simulink model "main_temp_new"  (R2021b)
settings: Solver=VariableStepAuto  StartTime=0.0  StopTime=50  RelTol=1e-3
model workspace (MAT data in the model file):
  op_trim2 : opcond.OperatingReport (value not decoded)
values from neighbouring files (symbols this model uses):
  ail = 8.316800428880180e-15    (= 8.31680042888e-15)    [lookupdata.m]
  CL = [  .0     .0     .0     .0     .0     .0     .0     .0     .0     .0     .0     .0 ... (first row only)    [lookupdata.m]
  CL2 = [ -.041  -.052  -.053  -.056  -.050  -.056  -.082  -.059  -.042  -.038  -.027  -.017 ... (first row only)    [lookupdata.m]
  CL3 = [ .005  .017  .014  .010  -.005  .009  .019  .005   .000  -.005  -.011  .008 ... (first row only)    [lookupdata.m]
  CLp = Damp(6,:)    [lookupdata.m]
  CLr = Damp(5,:)    [lookupdata.m]
  CM = [ .205   .168   .186   .196   .213   .251   .245   .238   .252   .231   .198   .192 ... (first row only)    [lookupdata.m]
  CMq = Damp(7,:)    [lookupdata.m]
  CN = [ .0    .0    .0    .0    .0    .0    .0    .0    .0     .0     .0     .0 ... (first row only)    [lookupdata.m]
  CN2 = [  .001  -.027  -.017  -.013  -.012  -.016   .001   .017   .011  .017   .008  .016 ... (first row only)    [lookupdata.m]
  CN3 = [ -.018  -.052  -.052  -.052  -.054  -.049  -.059  -.051  -.030  -.037  -.026  -.013 ... (first row only)    [lookupdata.m]
  CNp = Damp(9,:)    [lookupdata.m]
  CNr = Damp(8,:)    [lookupdata.m]
  CX = [ -0.0990   -0.0480   -0.0220   -0.0400   -0.0830 ... (first row only)    [lookupdata.m]
  CXq = Damp(1,:)    [lookupdata.m]
  CYp = Damp(3,:)    [lookupdata.m]
  CYr = Damp(2,:)    [lookupdata.m]
  CZ = [ 0.770  0.241  -0.100  -0.416  -0.731  -1.053  -1.366                                  -1.646  -1.917  -2.120  -2.248  -2.229 ]    [lookupdata.m]
  CZq = Damp(4,:)    [lookupdata.m]
  el = -2.205494777225563    (= -2.20549477723)    [lookupdata.m]
  Klqrlat = lqr(sys,Q,R)    [lat_lqr.m]
  Klqrlong = lqr(sys,Q,R)    [long_lqr.m]
  rud = -6.804083993307187e-14    (= -6.80408399331e-14)    [lookupdata.m]
  state_init = [ 598.9416 ; 0 ; 35.622639 ; 0 ; 0 ; 0 ;  0.01  ; 0.1 ;  0.1  ;        0 ; 0 ; 19950 ; 590 ; 0.059405952482911 ; 0 ; 15.941298293587984]    [lookupdata.m]
  th = 0.245477337443609    (= 0.245477337444)    [lookupdata.m]
  x_lat = [   0   ;     0    ;  0  ;  0  ; 0]    [lookupdata.m]
  x_long = [600 ; 20000 ; 0.059405952482911 ; 0.059405952482911 ; 0 ; 15.941298293587984]    [lookupdata.m]
undefined symbols (not defined in the file or in its folder): Earth, WGS84
libraries: simulink x4, aerolibfltsims x2, aerolibtransform2 x1, sldrtlib x1
settings Model: Creator=TecHNo-Pc  LastModifiedBy=TecHNo-Pc
settings SolverCC: AlgebraicLoopSolver=TrustRegion
settings DataIOCC: ExternalInput=getinputstruct(op_trim2)  InitialState=state_init  LoadInitialState=on
settings DebuggingCC: SFMachineParentedDataDiag=warning

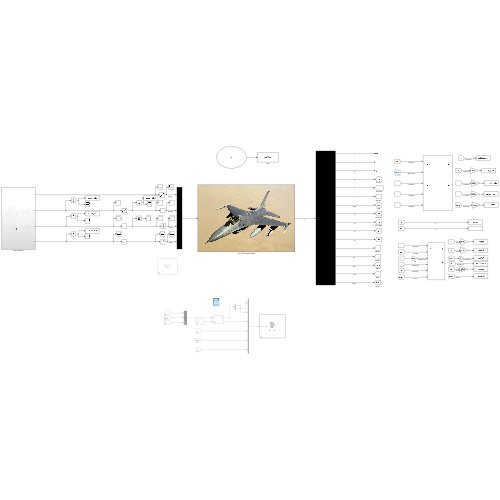
[thumbnail: Simulink's stored preview of the top-level diagram]
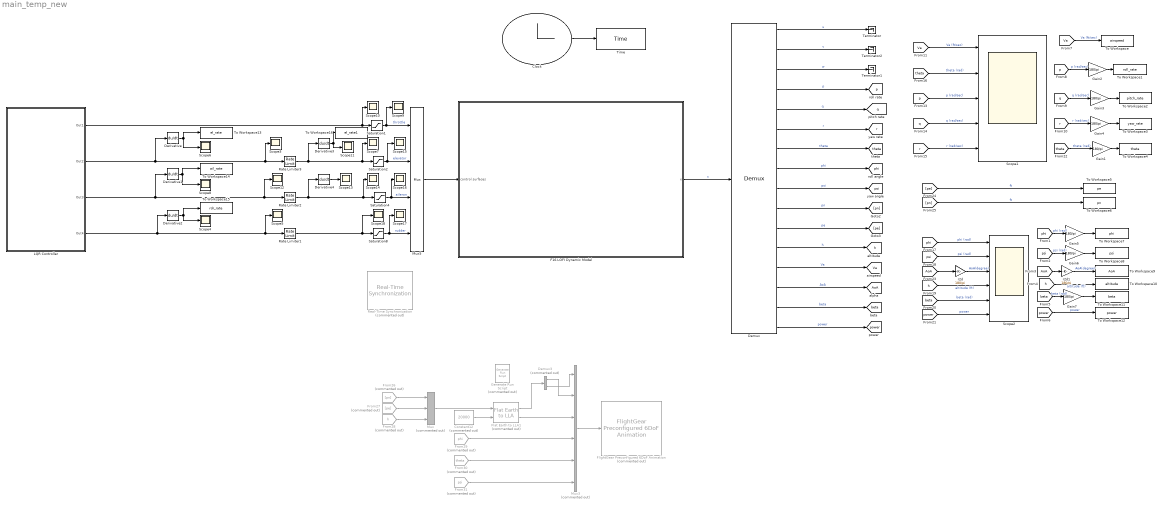
== system main_temp_new ==
  Clock : Clock
      settings: Decimation=50
  Constant12 : Constant  Commented=on  Value=20000
  Demux : Demux  Outputs=16
  Demux3 : Demux  Commented=on  Outputs=2
  Derivative{,1..4} (5 alike) : Derivative
  F16 LOFI Dynamic Model : Subsystem
      mask Display: image('$imagefile'); % Use "Edit Image" on toolstrip to change.
  Flat Earth to LLA1 : aerolibtransform2/Flat Earth to LLA  Commented=on  units=English  ptype=Earth (WGS84)  F=1/298.257223563  R=20925646.3255  refPosPort=off  LL0=[0 10]  psi=0
  FlightGear Preconfigured 6DoF Animation : aerolibfltsims/FlightGear Preconfigured 6DoF Animation  Commented=on  xFlightGearVersion=v2019.1  DestinationIpAddress=127.0.0.1  DestinationPort=5502  SampleTime=1/30  packetVersion=24
  From26 : From  Commented=on  GotoTag=pn
  From27 : From  Commented=on  GotoTag=pe
  From28 : From  Commented=on  GotoTag=h  TagVisibility=global
  From29 : From  Commented=on  GotoTag=phi  TagVisibility=global
  From30 : From  Commented=on  GotoTag=theta  TagVisibility=global
  From31 : From  Commented=on  GotoTag=psi  TagVisibility=global
  Gain{1..7} (7 alike) : Gain  Gain=180/pi
  Generate Run Script : aerolibfltsims/Generate Run Script  Commented=on  Architecture=Default  dataFlow=Send  GeometryModelName=c172p  AirportId=KSFO  RunwayId=10L  InitialAltitude=7224  InitialHeading=113  OffsetDistance=4.72  OffsetAzimuth=0  InstallScenery=off  DisableShaders=off  OriginAddress=127.0.0.1  DestinationPort=5502  OriginPort=5505  LocalAddress=127.0.0.1  OutputFileName=runfg.bat  FlightGearBaseDirectory=C:\Program Files\FlightGear 2020.3
  LQR Controller : Subsystem
  Mux : Mux  Commented=on  Inputs=3
  Mux3 : Mux  Commented=on  Inputs=6
  Mux5 : Mux
  Rate Limiter1 : RateLimiter  RisingSlewLimit=120  FallingSlewLimit=-120  SampleTimeMode=inherited
  Rate Limiter2 : RateLimiter  RisingSlewLimit=80  FallingSlewLimit=-80  SampleTimeMode=inherited
  Rate Limiter3 : RateLimiter  RisingSlewLimit=60  FallingSlewLimit=-60  SampleTimeMode=inherited
  Real-Time Synchronization : sldrtlib/Real-Time Synchronization  Commented=on  SampleTime=0.1  MaxMissedTicks=10  ShowMissedTicks=off  YieldWhenWaiting=off
  Saturation1 : Saturate  UpperLimit=1  LowerLimit=0
  Saturation2 : Saturate  UpperLimit=25  LowerLimit=-25
  Saturation4 : Saturate  UpperLimit=21.5  LowerLimit=-21.5
  Saturation8 : Saturate  UpperLimit=30  LowerLimit=-30
  Scope1 : Scope  NumInputPorts=5
  Scope{3..18} (16 alike) : Scope
  Scope2 : Scope  NumInputPorts=6
  Terminator : Terminator
  Terminator1 : Terminator
  Terminator2 : Terminator
  Time : ToWorkspace  VariableName=Time  SampleTime=-1
      settings: Decimation=100
  To Workspace : ToWorkspace  VariableName=airspeed  SampleTime=-1
  To Workspace1 : ToWorkspace  VariableName=roll_rate  SampleTime=-1
  To Workspace10 : ToWorkspace  VariableName=altitude  SampleTime=-1
  To Workspace11 : ToWorkspace  VariableName=beta  SampleTime=-1
  To Workspace12 : ToWorkspace  VariableName=power  SampleTime=-1
  To Workspace13 : ToWorkspace  VariableName=el_rate  SampleTime=-1
  To Workspace14 : ToWorkspace  VariableName=ail_rate  SampleTime=-1
  To Workspace15 : ToWorkspace  VariableName=rdr_rate  SampleTime=-1
  To Workspace16 : ToWorkspace  VariableName=el_rate1  SampleTime=-1
  To Workspace2 : ToWorkspace  VariableName=pitch_rate  SampleTime=-1
  To Workspace3 : ToWorkspace  VariableName=yaw_rate  SampleTime=-1
  To Workspace4 : ToWorkspace  VariableName=theta  SampleTime=-1
  To Workspace5 : ToWorkspace  VariableName=pe  SampleTime=-1
  To Workspace6 : ToWorkspace  VariableName=pn  SampleTime=-1
  To Workspace7 : ToWorkspace  VariableName=phi  SampleTime=-1
  To Workspace8 : ToWorkspace  VariableName=psi  SampleTime=-1
  To Workspace9 : ToWorkspace  VariableName=AoA  SampleTime=-1
  r2d : Gain  Gain=180/pi
  r2d1 : Gain  Gain=180/pi
  tag scope: AoA=global, Va=global, beta=global, h=global, p=global, phi=global, power=global, psi=global, q=global, r=global, theta=global
  wires:
  Demux/2 -> Terminator2/1  "v"
  Demux/3 -> Terminator1/1  "w"
  Demux/4 -> [p]  "p"
  Demux/6 -> [r]  "r"
  Demux/7 -> [theta]  "theta"
  Demux/8 -> [phi]  "phi"
  Demux/9 -> [psi]  "psi"
  Demux/10 -> [pn]  "pn"
  Demux/11 -> [pe]  "pe"
  Mux5/1 -> F16 LOFI Dynamic Model/1(control surfaces)
  Demux/13 -> [Va]  "Va"
  Demux/14 -> [AoA]  "AoA"
  Demux/15 -> [beta]  "beta"
  Demux/16 -> [power]  "power"
  Demux/1 -> Terminator/1  "u"
  Demux/5 -> [q]  "q"
  Demux/12 -> [h]  "h"
  F16 LOFI Dynamic Model/1(x) -> Demux/1  "x"
  [Va] -> Scope1/1  "Va (ft/sec)"
  [p] -> Scope1/3  "p (rad/sec)"
  [q] -> Scope1/4  "q (rad/sec)"
  [r] -> Scope1/5  "r (rad/sec)"
  [theta] -> Scope1/2  "theta (rad)"
  [phi] -> Scope2/1  "phi (rad)"
  [psi] -> Scope2/2  "psi (rad)"
  r2d/1 -> Scope2/3  "AoA(degree)"
  [h] -> Scope2/4  "altitude (ft)"
  [beta] -> Scope2/5  "beta (rad)"
  [power] -> Scope2/6  "power"
  [AoA] -> r2d/1
  [pe] -> To Workspace5/1  "ft"
  [pn] -> To Workspace6/1  "ft"
  Clock/1 -> Time/1
  Constant12/1 -> Flat Earth to LLA1/2
  Demux3/2 -> Mux3/1
  Demux3/1 -> Mux3/2
  Flat Earth to LLA1/1 -> Demux3/1
  Mux3/1 -> FlightGear Preconfigured 6DoF Animation/1
  Flat Earth to LLA1/2 -> Mux3/3
  Mux/1 -> Flat Earth to LLA1/1
  From26/1 -> Mux/1
  From27/1 -> Mux/2
  From28/1 -> Mux/3
  From29/1 -> Mux3/4
  From30/1 -> Mux3/5
  From31/1 -> Mux3/6
  Saturation2/1 -> Scope15/1, Mux5/2  "elevator"
  Saturation1/1 -> Scope9/1, Mux5/1  "throttle"
  Saturation4/1 -> Scope16/1, Mux5/3  "aileron"
  Saturation8/1 -> Scope17/1, Mux5/4  "rudder"
  LQR Controller/1(Out1) -> Saturation1/1, Scope10/1
  Gain1/1 -> To Workspace4/1
  Gain2/1 -> To Workspace1/1
  Gain3/1 -> To Workspace2/1
  Gain4/1 -> To Workspace3/1
  Gain5/1 -> To Workspace7/1
  Gain6/1 -> To Workspace8/1
  Gain7/1 -> To Workspace11/1
  Derivative/1 -> To Workspace13/1, Scope6/1
  LQR Controller/2(Out2) -> Rate Limiter3/1, Scope3/1, Derivative/1
  [phi] -> Gain5/1  "phi (rad)"
  [psi] -> Gain6/1  "psi (rad)"
  [AoA] -> r2d1/1
  r2d1/1 -> To Workspace9/1  "AoA(degree)"
  [beta] -> Gain7/1  "beta (rad)"
  [h] -> To Workspace10/1  "altitude (ft)"
  [power] -> To Workspace12/1  "power"
  [Va] -> To Workspace/1  "Va (ft/sec)"
  [p] -> Gain2/1  "p (rad/sec)"
  [q] -> Gain3/1  "q (rad/sec)"
  [r] -> Gain4/1  "r (rad/sec)"
  [theta] -> Gain1/1  "theta (rad)"
  Rate Limiter3/1 -> Derivative3/1, Scope7/1, Saturation2/1
  LQR Controller/3(Out3) -> Derivative1/1, Scope12/1, Rate Limiter2/1
  Derivative1/1 -> To Workspace14/1, Scope8/1
  Derivative2/1 -> To Workspace15/1, Scope4/1
  LQR Controller/4(Out4) -> Rate Limiter1/1, Scope5/1, Derivative2/1
  Rate Limiter1/1 -> Scope18/1, Saturation8/1
  Derivative3/1 -> To Workspace16/1, Scope11/1
  Derivative4/1 -> Scope13/1
  Rate Limiter2/1 -> Derivative4/1, Scope14/1, Saturation4/1

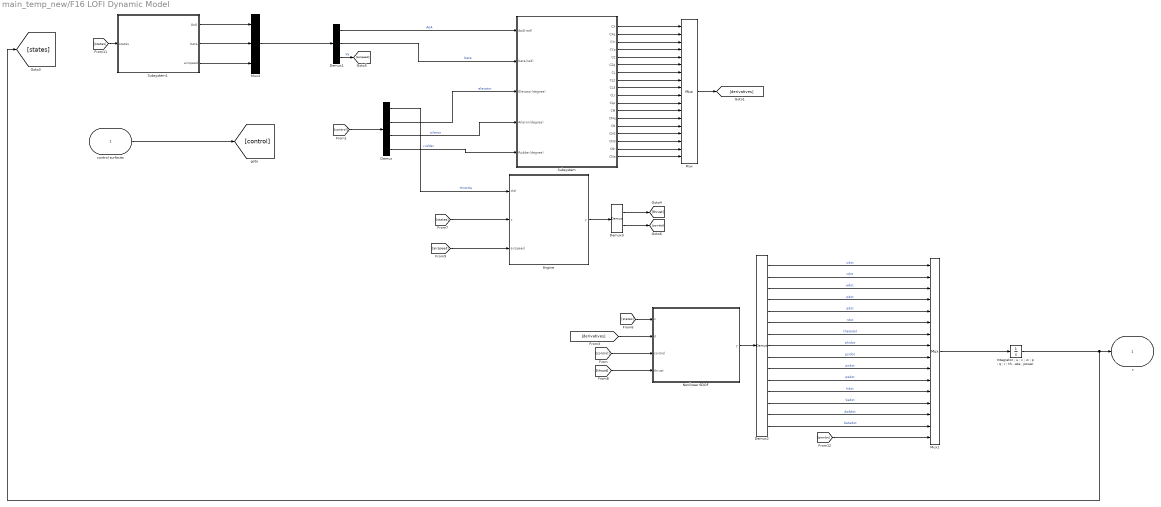
== system main_temp_new/F16 LOFI Dynamic Model ==
  control surfaces : Inport
  Demux : Demux
  Demux1 : Demux  Outputs=3
  Demux2 : Demux  Outputs=15
  Demux3 : Demux  Outputs=2
  Engine : MATLAB Function  TreatAsAtomicUnit=on
  Integrator ; u ; v ; w ; p ; q ; r ; theta ; phi ; psi ; pn ; pe ; h ; Va ; AoA ; beta ; power : Integrator  InitialCondition=state_init
  Mux : Mux  Inputs=18
  Mux1 : Mux  Inputs=16
  Mux4 : Mux  Inputs=3
  Nonlinear 6DOF : MATLAB Function  TreatAsAtomicUnit=on
  Subsystem : Subsystem
  Subsystem1 : Subsystem
  x : Outport
  wires:
  Subsystem/1(CX) -> Mux/1
  Subsystem/2(CXq) -> Mux/2
  Nonlinear 6DOF/1(y) -> Demux2/1
  Demux/2 -> Subsystem/3(Elevator(degree))  "elevator"
  Demux/1 -> Engine/1(thtl)  "throttle"
  Demux/3 -> Subsystem/4(Aileron(degree))  "aileron"
  Demux/4 -> Subsystem/5(Rudder(degree))  "rudder"
  Demux1/2 -> Subsystem/2(beta(rad))  "beta"
  Demux1/1 -> Subsystem/1(AoA(rad))  "AoA"
  Subsystem/3(CYr) -> Mux/3
  Subsystem/4(CYp) -> Mux/4
  Subsystem/5(CZ) -> Mux/5
  Subsystem/7(CL) -> Mux/7
  Demux1/3 -> [airspeed]  "Va"
  Demux2/2 -> Mux1/2  "vdot"
  Demux2/1 -> Mux1/1  "udot"
  Demux2/3 -> Mux1/3  "wdot"
  Demux2/5 -> Mux1/5  "qdot"
  Demux2/6 -> Mux1/6  "rdot"
  Demux2/7 -> Mux1/7  "thetadot"
  Demux2/8 -> Mux1/8  "phidot"
  Demux2/9 -> Mux1/9  "psidot"
  Demux2/10 -> Mux1/10  "pndot"
  Demux2/11 -> Mux1/11  "pedot"
  Demux2/12 -> Mux1/12  "hdot"
  control surfaces/1 -> [control]
  [control] -> Nonlinear 6DOF/3(control)
  [derivatives] -> Nonlinear 6DOF/2(d)
  Mux4/1 -> Demux1/1
  [control] -> Demux/1
  [states] -> Nonlinear 6DOF/1(x)
  [states] -> Engine/2(x)
  Engine/1(y) -> Demux3/1
  Demux3/1 -> [thrust]
  [thrust] -> Nonlinear 6DOF/4(thrust)
  [airspeed] -> Engine/3(airspeed)
  Subsystem/6(CZq) -> Mux/6
  Subsystem/8(CL2) -> Mux/8
  Subsystem/9(CL3) -> Mux/9
  Subsystem/10(CLr) -> Mux/10
  Subsystem/11(CLp) -> Mux/11
  Subsystem/12(CM) -> Mux/12
  Subsystem/13(CMq) -> Mux/13
  Subsystem/14(CN) -> Mux/14
  Subsystem/15(CN2) -> Mux/15
  Subsystem/16(CN3) -> Mux/16
  Subsystem/17(CNr) -> Mux/17
  Subsystem/18(CNp) -> Mux/18
  Mux/1 -> [derivatives]
  Subsystem1/1(AoA) -> Mux4/1
  Subsystem1/3(airspeed) -> Mux4/3
  Subsystem1/2(beta) -> Mux4/2
  [states] -> Subsystem1/1(states)
  Demux2/13 -> Mux1/13  "Vadot"
  Demux2/14 -> Mux1/14  "AoAdot"
  Demux2/15 -> Mux1/15  "betadot"
  Demux3/2 -> [powdot]
  Demux2/4 -> Mux1/4  "pdot"
  [powdot] -> Mux1/16
  Integrator ; u ; v ; w ; p ; q ; r ; theta ; phi ; psi ; pn ; pe ; h ; Va ; AoA ; beta ; power/1 -> x/1, [states]
  Mux1/1 -> Integrator ; u ; v ; w ; p ; q ; r ; theta ; phi ; psi ; pn ; pe ; h ; Va ; AoA ; beta ; power/1

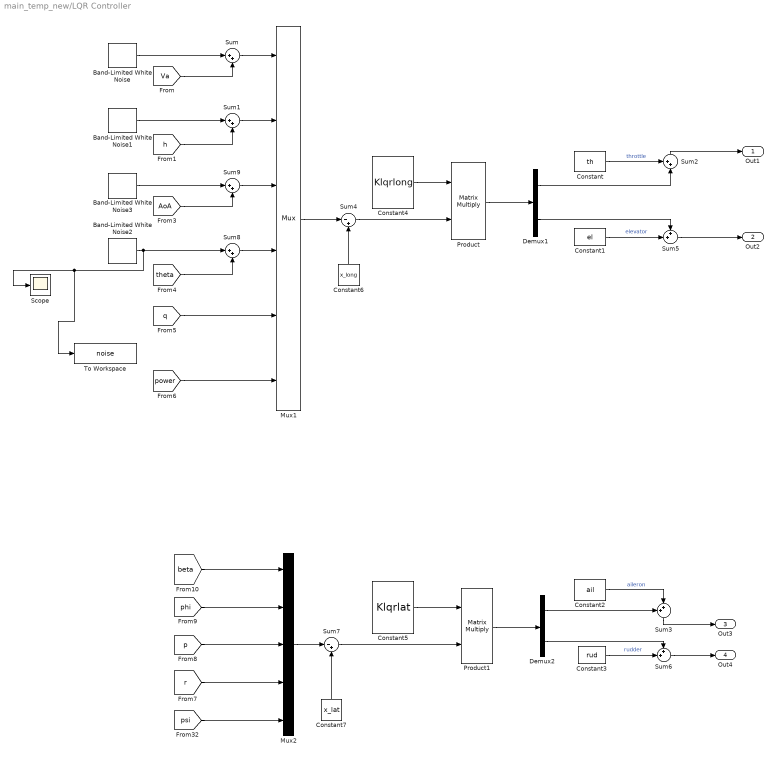
== system main_temp_new/LQR Controller ==
  Band-Limited White Noise : simulink/Sources/Band-Limited White Noise  Cov=0.1  Ts=0.1  seed=[23341]
  Band-Limited White Noise1 : simulink/Sources/Band-Limited White Noise  Cov=0.1  Ts=0.1  seed=[23341]
  Band-Limited White Noise2 : simulink/Sources/Band-Limited White Noise  Cov=0.00001  Ts=0.1  seed=[23341]
  Band-Limited White Noise3 : simulink/Sources/Band-Limited White Noise  Cov=0.00001  Ts=0.1  seed=[23341]
  Constant : Constant  Value=th
  Constant1 : Constant  Value=el
  Constant2 : Constant  Value=ail
  Constant3 : Constant  Value=rud
  Constant4 : Constant  Value=Klqrlong
  Constant5 : Constant  Value=Klqrlat
  Constant6 : Constant  Value=x_long
  Constant7 : Constant  Value=x_lat
  Demux1 : Demux  Outputs=2
  Demux2 : Demux  Outputs=2
  Mux1 : Mux  Inputs=6
  Mux2 : Mux  Inputs=5
  Product : Product  Multiplication=Matrix(*)
  Product1 : Product  Multiplication=Matrix(*)
  Scope : Scope
  Sum{,1,8..9} (4 alike) : Sum  Inputs=|++
  Sum{2..3,5..6} (4 alike) : Sum  Inputs=++|
  Sum4 : Sum  Inputs=|-+
  Sum7 : Sum  Inputs=|-+
  To Workspace : ToWorkspace  VariableName=noise  SampleTime=-1
  Out1 : Outport
  Out2 : Outport  Port=2
  Out3 : Outport  Port=3
  Out4 : Outport  Port=4
  wires:
  [theta] -> Sum8/2
  [q] -> Mux1/5
  [power] -> Mux1/6
  Demux1/1 -> Sum2/2
  Constant1/1 -> Sum5/2  "elevator"
  Product/1 -> Demux1/1
  [beta] -> Mux2/1
  Mux1/1 -> Sum4/1
  Sum2/1 -> Out1/1
  [Va] -> Sum/2
  [p] -> Mux2/3
  Constant4/1 -> Product/1
  Sum6/1 -> Out4/1
  [h] -> Sum1/2
  Constant2/1 -> Sum3/2  "aileron"
  [phi] -> Mux2/2
  Sum7/1 -> Product1/2
  Constant6/1 -> Sum4/2
  [psi] -> Mux2/5
  Mux2/1 -> Sum7/1
  Constant3/1 -> Sum6/2  "rudder"
  Demux2/2 -> Sum6/1
  Demux2/1 -> Sum3/1
  Demux1/2 -> Sum5/1
  Sum4/1 -> Product/2
  Constant/1 -> Sum2/1  "throttle"
  Product1/1 -> Demux2/1
  [r] -> Mux2/4
  Constant7/1 -> Sum7/2
  Sum5/1 -> Out2/1
  Constant5/1 -> Product1/1
  Sum3/1 -> Out3/1
  Band-Limited White Noise/1 -> Sum/1
  Sum/1 -> Mux1/1
  Sum1/1 -> Mux1/2
  Band-Limited White Noise1/1 -> Sum1/1
  [AoA] -> Sum9/2
  Band-Limited White Noise2/1 -> To Workspace/1, Scope/1, Sum8/1
  Sum8/1 -> Mux1/4
  Band-Limited White Noise3/1 -> Sum9/1
  Sum9/1 -> Mux1/3

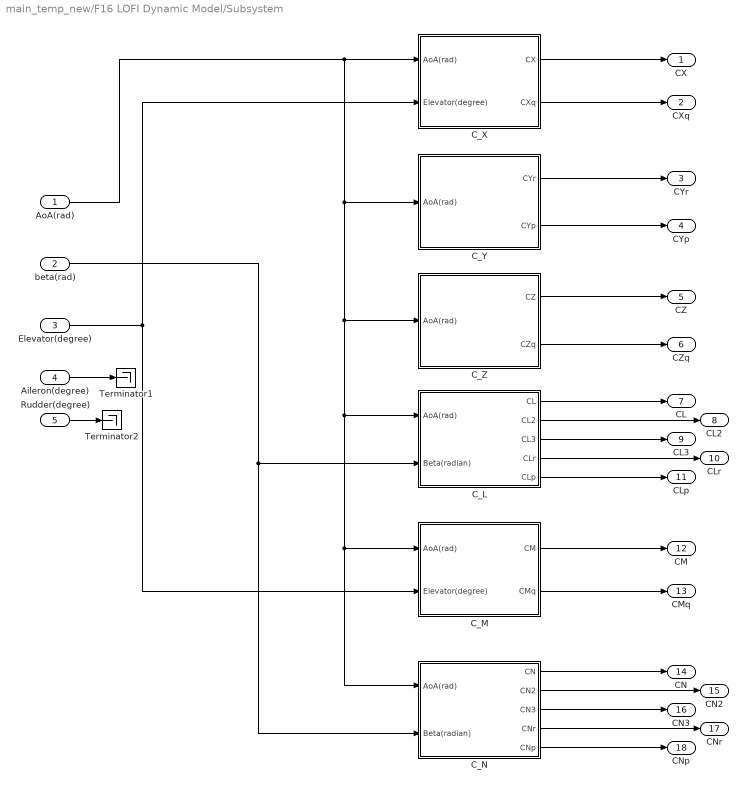
== system main_temp_new/F16 LOFI Dynamic Model/Subsystem ==
  AoA(rad) : Inport
  beta(rad) : Inport  Port=2
  Elevator(degree) : Inport  Port=3
  Aileron(degree) : Inport  Port=4
  Rudder(degree) : Inport  Port=5
  C_L : Subsystem
  C_M : Subsystem
  C_N : Subsystem
  C_X : Subsystem
  C_Y : Subsystem
  C_Z : Subsystem
  Terminator1 : Terminator
  Terminator2 : Terminator
  CX : Outport
  CXq : Outport  Port=2
  CYr : Outport  Port=3
  CYp : Outport  Port=4
  CZ : Outport  Port=5
  CZq : Outport  Port=6
  CL : Outport  Port=7
  CL2 : Outport  Port=8
  CL3 : Outport  Port=9
  CLr : Outport  Port=10
  CLp : Outport  Port=11
  CM : Outport  Port=12
  CMq : Outport  Port=13
  CN : Outport  Port=14
  CN2 : Outport  Port=15
  CN3 : Outport  Port=16
  CNr : Outport  Port=17
  CNp : Outport  Port=18
  wires:
  C_X/1(CX) -> CX/1
  C_X/2(CXq) -> CXq/1
  C_Y/1(CYr) -> CYr/1
  C_Y/2(CYp) -> CYp/1
  C_Z/1(CZ) -> CZ/1
  C_L/1(CL) -> CL/1
  C_L/4(CLr) -> CLr/1
  C_L/5(CLp) -> CLp/1
  C_M/1(CM) -> CM/1
  C_M/2(CMq) -> CMq/1
  C_N/1(CN) -> CN/1
  C_N/5(CNp) -> CNp/1
  C_N/4(CNr) -> CNr/1
  AoA(rad)/1 -> C_N/1(AoA(rad)), C_M/1(AoA(rad)), C_L/1(AoA(rad)), C_Z/1(AoA(rad)), C_Y/1(AoA(rad)), C_X/1(AoA(rad))
  Elevator(degree)/1 -> C_X/2(Elevator(degree)), C_M/2(Elevator(degree))
  Aileron(degree)/1 -> Terminator1/1
  Rudder(degree)/1 -> Terminator2/1
  C_Z/2(CZq) -> CZq/1
  C_L/2(CL2) -> CL2/1
  C_L/3(CL3) -> CL3/1
  C_N/2(CN2) -> CN2/1
  C_N/3(CN3) -> CN3/1
  beta(rad)/1 -> C_N/2(Beta(radian)), C_L/2(Beta(radian))

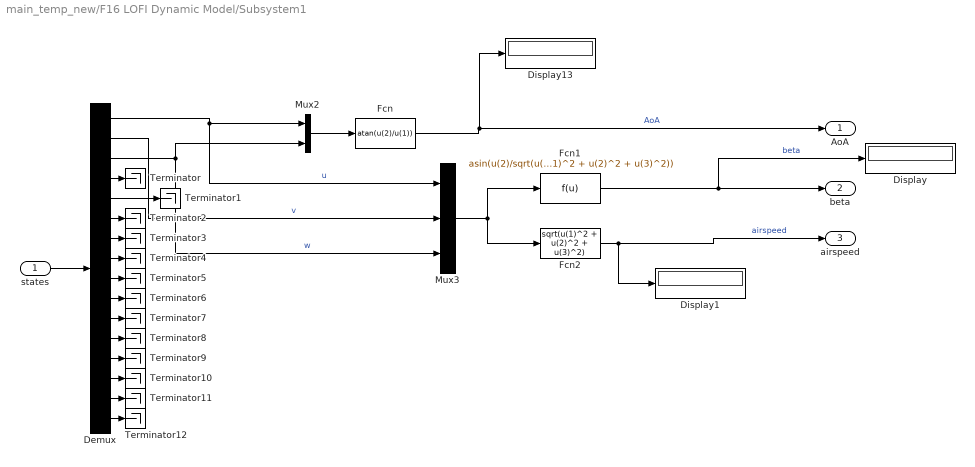
== system main_temp_new/F16 LOFI Dynamic Model/Subsystem1 ==
  states : Inport
  Demux : Demux  Outputs=16
  Display : Display
  Display1 : Display
  Display13 : Display
  Fcn : Fcn  Expr=atan(u(2)/u(1))
  Fcn1 : Fcn  Expr=asin(u(2)/sqrt(u(1)^2 + u(2)^2 + u(3)^2))
  Fcn2 : Fcn  Expr=sqrt(u(1)^2 + u(2)^2 + u(3)^2)
  Mux2 : Mux  Inputs=2
  Mux3 : Mux  Inputs=3
  Terminator{,1..12} (13 alike) : Terminator
  AoA : Outport
  beta : Outport  Port=2
  airspeed : Outport  Port=3
  wires:
  Mux3/1 -> Fcn2/1, Fcn1/1
  Fcn/1 -> Display13/1, AoA/1  "AoA"
  Mux2/1 -> Fcn/1
  Fcn2/1 -> Display1/1, airspeed/1  "airspeed"
  Fcn1/1 -> Display/1, beta/1  "beta"
  states/1 -> Demux/1
  Demux/1 -> Mux3/1, Mux2/1  "u"
  Demux/3 -> Mux3/3, Mux2/2  "w"
  Demux/2 -> Mux3/2  "v"
  Demux/11 -> Terminator7/1
  Demux/10 -> Terminator6/1
  Demux/9 -> Terminator5/1
  Demux/8 -> Terminator4/1
  Demux/7 -> Terminator3/1
  Demux/6 -> Terminator2/1
  Demux/5 -> Terminator1/1
  Demux/4 -> Terminator/1
  Demux/12 -> Terminator8/1
  Demux/13 -> Terminator9/1
  Demux/14 -> Terminator10/1
  Demux/15 -> Terminator11/1
  Demux/16 -> Terminator12/1

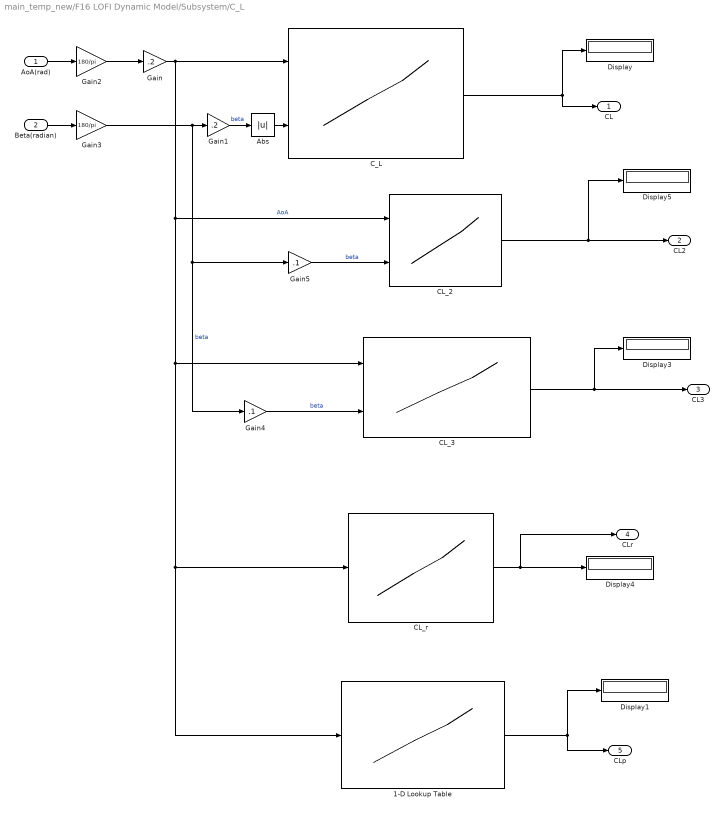
== system main_temp_new/F16 LOFI Dynamic Model/Subsystem/C_L ==
  AoA(rad) : Inport
  Beta(radian) : Inport  Port=2
  1-D Lookup Table : Lookup_n-D  NumberOfTableDimensions=1  BreakpointsForDimension1=[-2:9]  Table=CLp  InternalRulePriority=Speed  RndMeth=Simplest  InputSameDT=on
  Abs : Abs
  CL_2 : Lookup_n-D  BreakpointsForDimension1=[-2:9]  BreakpointsForDimension2=[-3:3]  Table=CL2  InternalRulePriority=Speed  RndMeth=Simplest  InputSameDT=on
      settings: InputPortMap=u0,u1
  CL_3 : Lookup_n-D  BreakpointsForDimension1=[-2:9]  BreakpointsForDimension2=[-3:3]  Table=CL3  InternalRulePriority=Speed  RndMeth=Simplest  InputSameDT=on
      settings: InputPortMap=u0,u1
  CL_r : Lookup_n-D  NumberOfTableDimensions=1  BreakpointsForDimension1=[-2:9]  Table=CLr  InternalRulePriority=Speed  RndMeth=Simplest  InputSameDT=on
  C_L : Lookup_n-D  BreakpointsForDimension1=[-2:9]  BreakpointsForDimension2=[0:6]  Table=CL  InternalRulePriority=Speed  RndMeth=Simplest  InputSameDT=on
      settings: InputPortMap=u0,u1
  Display{,1,3..5} (5 alike) : Display
  Gain : Gain  Gain=.2
  Gain1 : Gain  Gain=.2
  Gain2 : Gain  Gain=180/pi
  Gain3 : Gain  Gain=180/pi
  Gain4 : Gain  Gain=.1
  Gain5 : Gain  Gain=.1
  CL : Outport
  CL2 : Outport  Port=2
  CL3 : Outport  Port=3
  CLr : Outport  Port=4
  CLp : Outport  Port=5
  wires:
  Gain3/1 -> Gain1/1, Gain5/1, Gain4/1  "beta"
  Gain/1 -> CL_2/1, 1-D Lookup Table/1, CL_r/1, CL_3/1, C_L/1  "AoA"
  AoA(rad)/1 -> Gain2/1
  Gain2/1 -> Gain/1
  Beta(radian)/1 -> Gain3/1
  C_L/1 -> CL/1, Display/1
  CL_2/1 -> Display5/1, CL2/1
  CL_3/1 -> CL3/1, Display3/1
  CL_r/1 -> Display4/1, CLr/1
  1-D Lookup Table/1 -> CLp/1, Display1/1
  Abs/1 -> C_L/2
  Gain1/1 -> Abs/1  "beta"
  Gain4/1 -> CL_3/2  "beta"
  Gain5/1 -> CL_2/2  "beta"

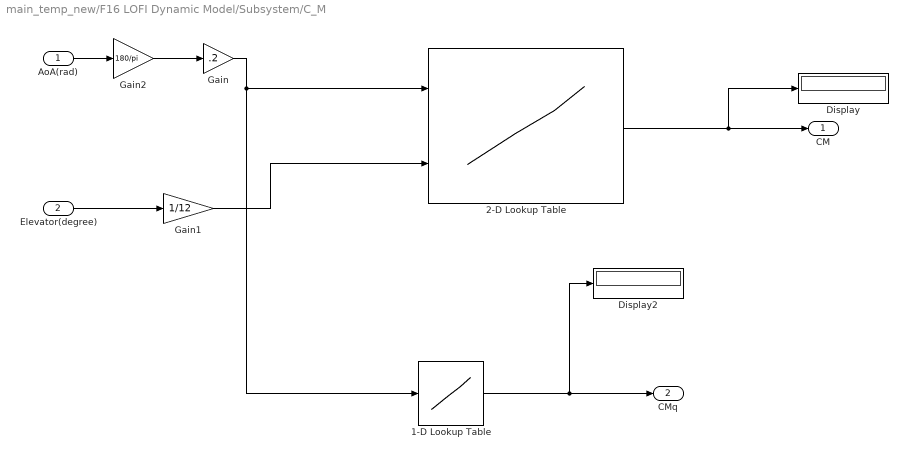
== system main_temp_new/F16 LOFI Dynamic Model/Subsystem/C_M ==
  AoA(rad) : Inport
  Elevator(degree) : Inport  Port=2
  1-D Lookup Table : Lookup_n-D  NumberOfTableDimensions=1  BreakpointsForDimension1=[-2:9]  Table=CMq  InternalRulePriority=Speed  RndMeth=Simplest  InputSameDT=on
  2-D Lookup Table : Lookup_n-D  BreakpointsForDimension1=[-2:9]  BreakpointsForDimension2=[-2:2]  Table=CM  InternalRulePriority=Speed  RndMeth=Simplest  InputSameDT=on
      settings: InputPortMap=u0,u1
  Display : Display
  Display2 : Display
  Gain : Gain  Gain=.2
  Gain1 : Gain  Gain=1/12
  Gain2 : Gain  Gain=180/pi
  CM : Outport
  CMq : Outport  Port=2
  wires:
  Gain1/1 -> 2-D Lookup Table/2
  Gain/1 -> 2-D Lookup Table/1, 1-D Lookup Table/1
  AoA(rad)/1 -> Gain2/1
  Gain2/1 -> Gain/1
  Elevator(degree)/1 -> Gain1/1
  2-D Lookup Table/1 -> Display/1, CM/1
  1-D Lookup Table/1 -> CMq/1, Display2/1

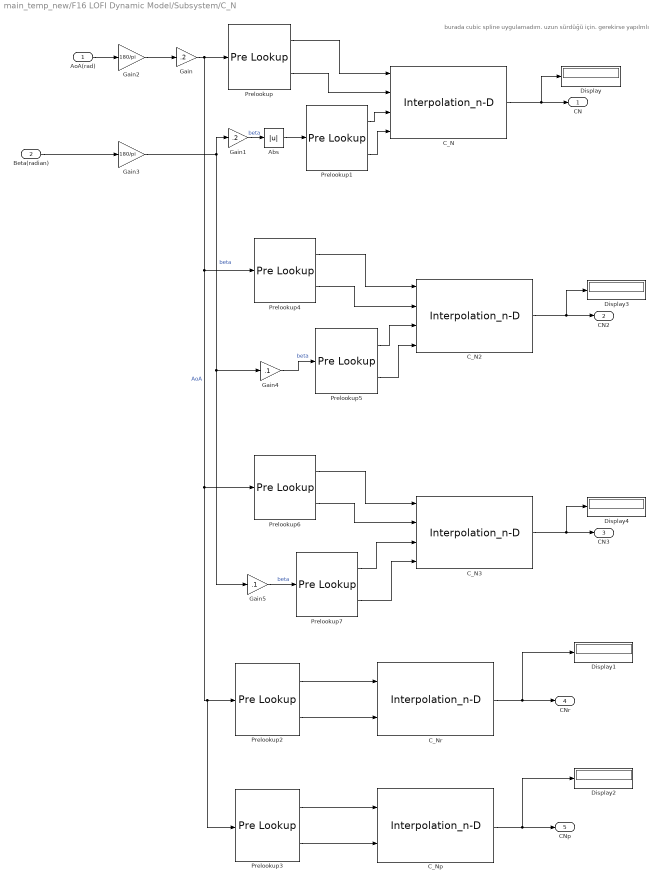
== system main_temp_new/F16 LOFI Dynamic Model/Subsystem/C_N ==
  note: burada cubic spline uygulamadım. uzun sürdüğü için. gerekirse yapılmlı
  AoA(rad) : Inport
  Beta(radian) : Inport  Port=2
  Abs : Abs
  C_N : Interpolation_n-D  Table=CN  InternalRulePriority=Speed
  C_N2 : Interpolation_n-D  Table=CN2  InternalRulePriority=Speed
  C_N3 : Interpolation_n-D  Table=CN3  InternalRulePriority=Speed
  C_Np : Interpolation_n-D  NumberOfTableDimensions=1  Table=CNp  InternalRulePriority=Speed
      settings: InputPortMap=u0,u1
  C_Nr : Interpolation_n-D  NumberOfTableDimensions=1  Table=CNr  InternalRulePriority=Speed
      settings: InputPortMap=u0,u1
  Display{,1..4} (5 alike) : Display
  Gain : Gain  Gain=.2
  Gain1 : Gain  Gain=.2
  Gain2 : Gain  Gain=180/pi
  Gain3 : Gain  Gain=180/pi
  Gain4 : Gain  Gain=.1
  Gain5 : Gain  Gain=.1
  Prelookup{,2..4,6} (5 alike) : PreLookup  BreakpointsData=AoA  ExtrapMethod=Linear
  Prelookup1 : PreLookup  BreakpointsData=beta  ExtrapMethod=Linear
  Prelookup5 : PreLookup  BreakpointsData=[-3:3]  ExtrapMethod=Linear
  Prelookup7 : PreLookup  BreakpointsData=[-3:3]  ExtrapMethod=Linear
  CN : Outport
  CN2 : Outport  Port=2
  CN3 : Outport  Port=3
  CNr : Outport  Port=4
  CNp : Outport  Port=5
  wires:
  Prelookup/1 -> C_N/1
  Prelookup1/2 -> C_N/4
  Gain3/1 -> Gain5/1, Gain4/1, Gain1/1  "beta"
  Prelookup/2 -> C_N/2
  Gain/1 -> Prelookup4/1, Prelookup6/1, Prelookup3/1, Prelookup2/1, Prelookup/1  "AoA"
  AoA(rad)/1 -> Gain2/1
  Prelookup1/1 -> C_N/3
  Gain2/1 -> Gain/1
  Beta(radian)/1 -> Gain3/1
  Prelookup2/2 -> C_Nr/2
  C_Nr/1 -> Display1/1, CNr/1
  Prelookup2/1 -> C_Nr/1
  C_N/1 -> Display/1, CN/1
  Prelookup3/1 -> C_Np/1
  C_Np/1 -> Display2/1, CNp/1
  Prelookup3/2 -> C_Np/2
  C_N2/1 -> Display3/1, CN2/1
  Prelookup4/1 -> C_N2/1
  Prelookup5/2 -> C_N2/4
  Prelookup5/1 -> C_N2/3
  Prelookup4/2 -> C_N2/2
  C_N3/1 -> Display4/1, CN3/1
  Prelookup6/1 -> C_N3/1
  Prelookup7/2 -> C_N3/4
  Prelookup7/1 -> C_N3/3
  Prelookup6/2 -> C_N3/2
  Abs/1 -> Prelookup1/1
  Gain1/1 -> Abs/1  "beta"
  Gain4/1 -> Prelookup5/1  "beta"
  Gain5/1 -> Prelookup7/1  "beta"

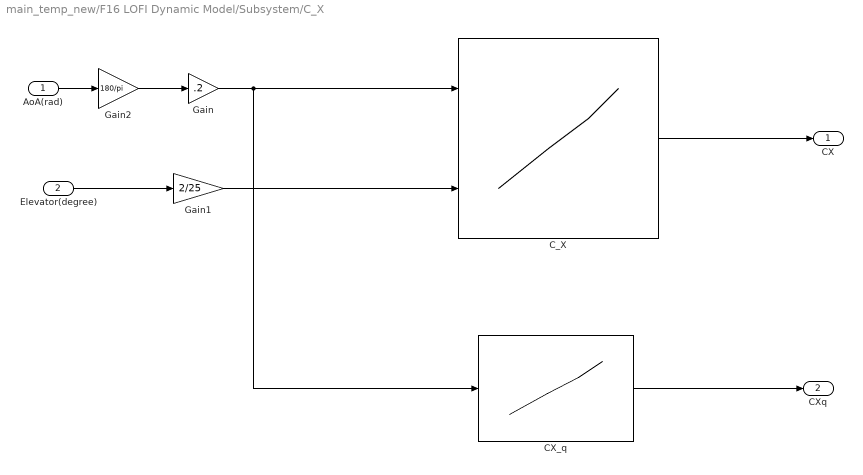
== system main_temp_new/F16 LOFI Dynamic Model/Subsystem/C_X ==
  AoA(rad) : Inport
  Elevator(degree) : Inport  Port=2
  CX_q : Lookup_n-D  NumberOfTableDimensions=1  BreakpointsForDimension1=[-2:9]  Table=CXq  InternalRulePriority=Speed  RndMeth=Simplest  InputSameDT=on
  C_X : Lookup_n-D  BreakpointsForDimension1=[-2:9]  BreakpointsForDimension2=[-2:2]  Table=CX  InternalRulePriority=Speed  RndMeth=Simplest  InputSameDT=on
      settings: InputPortMap=u0,u1
  Gain : Gain  Gain=.2
  Gain1 : Gain  Gain=2/25
  Gain2 : Gain  Gain=180/pi
  CX : Outport
  CXq : Outport  Port=2
  wires:
  Gain1/1 -> C_X/2
  Gain/1 -> CX_q/1, C_X/1
  AoA(rad)/1 -> Gain2/1
  Gain2/1 -> Gain/1
  Elevator(degree)/1 -> Gain1/1
  CX_q/1 -> CXq/1
  C_X/1 -> CX/1

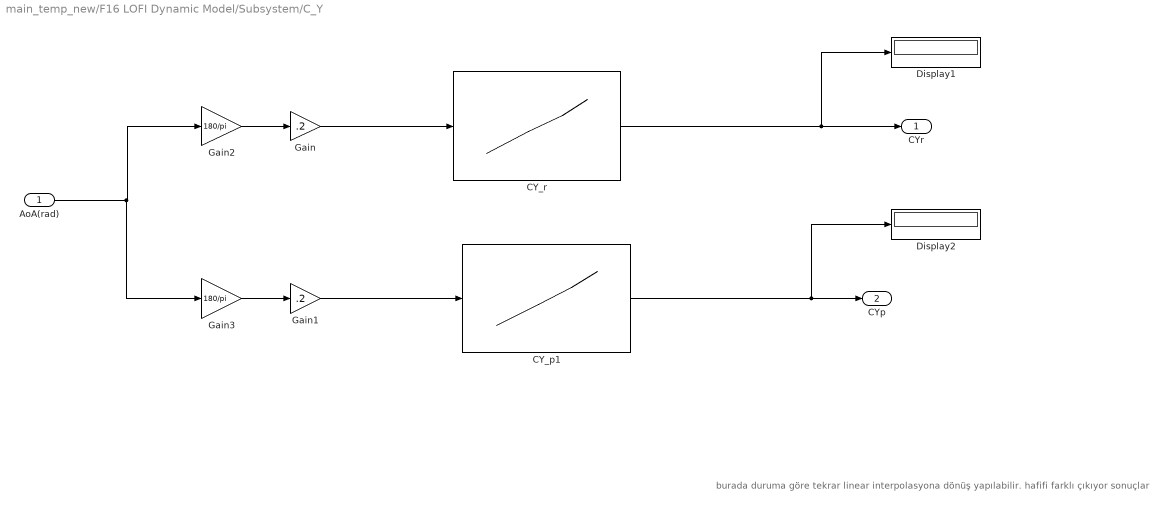
== system main_temp_new/F16 LOFI Dynamic Model/Subsystem/C_Y ==
  note: burada duruma göre tekrar linear interpolasyona dönüş yapılabilir. hafifi farklı çıkıyor sonuçlar
  AoA(rad) : Inport
  CY_p1 : Lookup_n-D  NumberOfTableDimensions=1  BreakpointsForDimension1=[-2:9]  Table=CYp  InternalRulePriority=Speed  RndMeth=Simplest  InputSameDT=on
  CY_r : Lookup_n-D  NumberOfTableDimensions=1  BreakpointsForDimension1=[-2:9]  Table=CYr  InternalRulePriority=Speed  RndMeth=Simplest  InputSameDT=on
  Display1 : Display
  Display2 : Display
  Gain : Gain  Gain=.2
  Gain1 : Gain  Gain=.2
  Gain2 : Gain  Gain=180/pi
  Gain3 : Gain  Gain=180/pi
  CYr : Outport
  CYp : Outport  Port=2
  wires:
  Gain/1 -> CY_r/1
  Gain2/1 -> Gain/1
  CY_p1/1 -> CYp/1, Display2/1
  Gain3/1 -> Gain1/1
  AoA(rad)/1 -> Gain3/1, Gain2/1
  CY_r/1 -> Display1/1, CYr/1
  Gain1/1 -> CY_p1/1

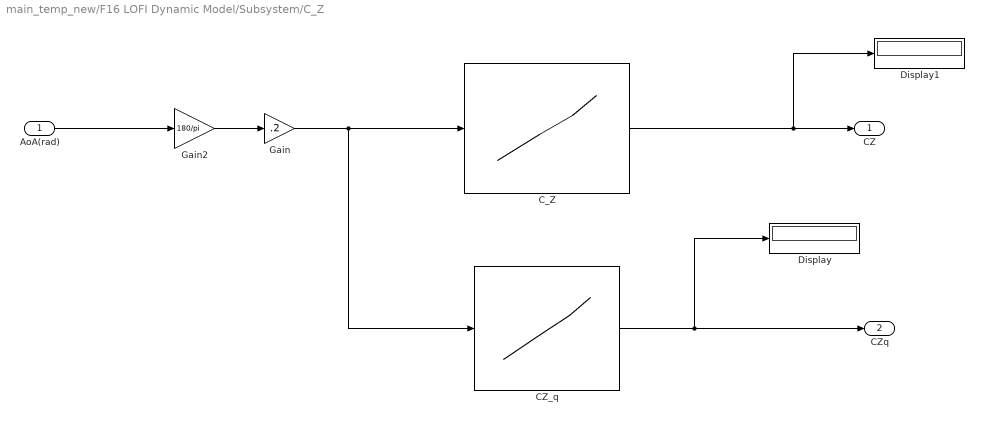
== system main_temp_new/F16 LOFI Dynamic Model/Subsystem/C_Z ==
  AoA(rad) : Inport
  CZ_q : Lookup_n-D  NumberOfTableDimensions=1  BreakpointsForDimension1=[-2:9]  Table=CZq  InternalRulePriority=Speed  RndMeth=Simplest  InputSameDT=on
  C_Z : Lookup_n-D  NumberOfTableDimensions=1  BreakpointsForDimension1=[-2:9]  Table=CZ  InternalRulePriority=Speed  RndMeth=Simplest  InputSameDT=on
  Display : Display
  Display1 : Display
  Gain : Gain  Gain=.2
  Gain2 : Gain  Gain=180/pi
  CZ : Outport
  CZq : Outport  Port=2
  wires:
  Gain/1 -> CZ_q/1, C_Z/1
  Gain2/1 -> Gain/1
  C_Z/1 -> Display1/1, CZ/1
  AoA(rad)/1 -> Gain2/1
  CZ_q/1 -> Display/1, CZq/1

== matlab function main_temp_new/F16 LOFI Dynamic Model/Engine ==
  data: thtl input; y output; x input; airspeed input
function y = fcn(thtl,x,airspeed)


if ( thtl <= 0.77 )
    tgear_value = 64.94 * thtl;
else
    tgear_value = 217.38 * thtl - 117.38;
end


%% cpow = power level command, percent
cpow = tgear_value;

%% pow = engine power level, percent
pow = x(16);

function  tau_r = rtau ( dp )

if ( dp <= 25.0 )
    tau_r = 1.0;  %%  reciprocal time constant 
elseif ( dp >= 50.0 )
        tau_r = 0.1;
else
    tau_r = 1.9 - 0.036 * dp;
end
end



if ( cpow >= 50.0 )
    if ( pow >= 50.0)
        tpow = cpow;
        t = 5.0;
    else
        tpow = 60.0;
        t = rtau ( tpow - pow );
    end
else
    if ( pow >= 50.0)
        tpow = 40.0;
        t = 5.0;
    else
        tpow = cpow;
        t = rtau ( tpow - pow );
    end
end 

% buradaki t ara değişken. sıcaklık veya thrust değil muhtemelen
power_dot = t * ( tpow - pow );


Va = airspeed;%ft/s



alt = x(12); 
r0 = 2.37764e-3;  % const, sea-level density, slugs/ft^3

tfac = 1.0 - 0.703e-5 * alt;
T = 519.0 * tfac;  % temperature, Rankine scale

if ( alt >= 35000.0 )
    T = 390.0;
end
rho = r0 * ( tfac ^ 4.14 );  % density
rmach = Va / sqrt ( 1.4 * 1716.3 * T ); % Mach number





% A - idle
% B - military
% C - maximum

A = [  1060.0    670.0     880.0    1140.0  1500.0   1860.0; 
       635.0     425.0     690.0    1010.0  1330.0   1700.0;
        60.0     25.0      345.0     755.0  1130.0   1525.0;
      -1020.0    -710.0   -300.0     350.0   910.0   1360.0;
      -2700.0   -1900.0   -1300.0   -247.0   600.0   1100.0;
      -3600.0   -1400.0   -595.0    -342.0  -200.0    700.0 ];
A = A';  
  
B = [ 12680.0  9150.0    6200.0   3950.0   2450.0   1400.0;
      12680.0  9150.0    6313.0   4040.0   2470.0   1400.0;
      12610.0  9312.0    6610.0   4290.0   2600.0   1560.0;
      12640.0  9839.0    7090.0   4660.0   2840.0   1660.0;
      12390.0  10176.0   7750.0   5320.0   3250.0   1930.0;
      11680.0  9848.0    8050.0   6100.0   3800.0   2310.0 ];
B = B';  

C = [ 20000.0  15000.0  10800.0   7000.0   4000.0   2500.0;
      21420.0  15700.0  11225.0   7323.0   4435.0   2600.0;
      22700.0  16860.0  12250.0   8154.0   5000.0   2835.0;
      24240.0  18910.0  13760.0   9285.0   5700.0   3215.0;
      26070.0  21075.0  15975.0  11115.0   6860.0   3950.0;
      28886.0  23319.0  18300.0  13484.0   8642.0   5057.0 ];  
C = C';  

row = 1;
col = 1;

h = 0.0001 * alt;
i = fix( h );
if (i >= 5)
    i = 4;
elseif (i <= 0)
     i = 0;
end
dh = h - i;
rm = 5.0 * rmach;
%  disp('rmach'); rmach
m = fix( rm );
if ( m >= 5 )
    m = 4;
elseif (m <= 0)
     m = 0;
end
dm = rm - m;
cdh = 1.0 - dh;
%  disp('i+row'); i+row
%  disp('m+row'); m+row
s = B( i+row, m+col ) * cdh + B( i+1+row, m+col ) * dh;
t = B( i+row, m+1+col ) * cdh + B( i+1+row, m+1+col ) * dh;
tmil = s + ( t - s ) * dm;
if( pow < 50.0 )
    s = A( i+row, m+col )   * cdh + A( i+1+row, m+col ) * dh;
    t = A( i+row, m+1+col ) * cdh + A( i+1+row, m+1+col ) * dh;
    tidl = s + ( t - s ) * dm;
    thrust_value = tidl + ( tmil - tidl ) * pow *0.02;
else
    s = C( i+row, m+col )   * cdh + C( i+1+row, m+col ) * dh;
    t = C( i+row, m+1+col ) * cdh + C( i+1+row, m+1+col ) * dh;
    tmax = s + ( t - s ) * dm;
    thrust_value = tmil + ( tmax - tmil ) * ( pow - 50.0 ) * 0.02;
end

y = [thrust_value  power_dot];

end

== matlab function main_temp_new/F16 LOFI Dynamic Model/Nonlinear 6DOF ==
  data: x input; y output; d input; control input; thrust input
function y = fcn(x,d,control,thrust)
    % x = [u v w p q r theta phi psi pn pe h V AoA(radian) beta(radian) power]
    % d = [CX CXq CYr CYp CZ CL CLr CLp CM CMq CN CNr CNp]
    % c = [throttle elevator(degree) aileron(degree) rudder(degree)]
    % isa = [T(K) a(m/s) p(Pa) rho(kg/m3)]



%%  constant variable
s = 300;
b = 30;
cbar = 11.32;
m = 636.9427;
xcgr = 0.35;
he = 160.0;
g = 32.174;

%% Inertia constants
c1 = -0.770;
c2 = 0.02755;
c3 = 1.055e-4;
c4 = 1.642e-6;
c5 = 0.9604;
c6 = 1.759e-2;
c7 = 1.792e-5;
c8 = -0.7336;
c9 = 1.587e-5;



%%  Assign state variables 

Va = x(13);
alpha = x(14);
beta = x(15);
phi = x(8);
theta = x(7);
psi = x(9);
p = x(4);
q = x(5);
r = x(6);



%%  Assign state & control variables 
throttle = control(1);
elevator   = control(2);
aileron  = control(3);
rudder  = control(4);

%% Air Data computer and engine model 

t = thrust;

h = x(12);
rho = 2.377e-03*(1-0.703e-05*h)^(4.14);

qbar = 0.5*rho*Va^2;

%% Look-up tables and component biuldup 

    CX = d(1) ;
    CXq = d(2) ;
    CY = (-0.02*beta*57.3 + 0.021*aileron/20 + 0.086*rudder/30);
    CYr = d(3);
    CYp = d(4) ;
    CZ = d(5);
    CZq = d(6) ;
    
    CL = d(7);
    CL2 = d(8);
    CL3 = d(9);
    CLr = d(10) ;
    CLp = d(11) ;
    
    CM = d(12);
    CMq = d(13); 
    CN = d(14);
    CN2 = d(15) ; 
    CN3 = d(16); 
    CNr = d(17);
    CNp = d(18);
    
            
    if beta<0
        CL = -CL;
        CN = -CN;
    end
    
%%  Add damping derivatives 

cxt = CX + cbar/(2*Va)*q*CXq;

cyt = CY + b/(2*Va)*(r*CYr + p*CYp);

czt = CZ*(1-(beta/57.3)^2) - 0.19*(elevator/25) + cbar/(2*Va)*q*CZq;

clt = CL + b/(2*Va)*(CLr*r+CLp*p) + CL2*aileron/20 + CL3*rudder/30;

xcg = 0.3;
cmt = CM + cbar/(2*Va)*CMq*q + czt*(0.35-xcg);


cnt = CN + b/(2*Va)*(CNr*r + CNp*p) - cbar/b*cyt*(xcgr-xcg)+CN2*aileron/20 + CN3*rudder/30 ;

%% Translational

u = Va * cos( alpha ) * cos( beta );
v = Va * sin( beta );
w = Va * sin( alpha ) * cos( beta );

sth = sin( theta );
cth = cos( theta );
sph = sin( phi );
cph = cos( phi );
spsi = sin( psi );
cpsi = cos( psi );


udot = r * v - q * w - g * sth + ( qbar * s * cxt + t )/m;
vdot = p * w - r * u + g * cth * sph + qbar * s/m * cyt;
wdot = q * u - p * v + g * cth * cph + qbar * s/m * czt;
  


Vadot = ( u * udot + v * vdot + w * wdot ) / Va;
AoAdot = (u * wdot - w * udot ) / ( u * u + w * w );
betadot = (Va * vdot - v * Va ) * cos( beta ) / ( u * u + w * w );

%% Attitudes
phidot = p + ( sth / cth ) * (q * sph + r * cph );
thetadot = q * cph - r * sph;
psidot = ( q * sph + r * cph ) / cth;

%% Rotational velocity
pdot = ( c2 * p + c1 * r + c4 * he ) * q + qbar * s * b * ( c3 * clt + c4 * cnt );

qdot = ( c5 * p -c7 * he )* r + c6 * ( r^2 - p^2 ) + qbar * s * cbar * c7 * cmt;
rdot = ( c8 * p - c2 * r + c9 * he ) * q + qbar * s * b * ( c4 * clt + c9 * cnt );

%% Navigation 

pndot = u * cth * cpsi + v * sph * cpsi * sth - cph * spsi + w * cph * sth * cpsi +sph * spsi;  %% north speed
pedot = u * cth * spsi + v * sph * spsi * sth + cph * cpsi + w * cph * sth * spsi - sph * cpsi;  %% east speed
hdot = u * sth - v * sph * cth - w * cph * cth; %% vertical speed



%% Outputs 

y = [udot ; vdot ; wdot ; pdot ; qdot ; rdot ; thetadot ; phidot ;...
            psidot ; pndot ; pedot ; hdot ; Vadot ; AoAdot ; betadot];
